simulink model "Frida"  (R2024b)
settings: Solver=VariableStepAuto  StartTime=0.0  StopTime=10.0  RelTol=1e-3
settings DataIOCC: SaveTime=off  ReturnWorkspaceOutputs=off  TimeSaveName=t

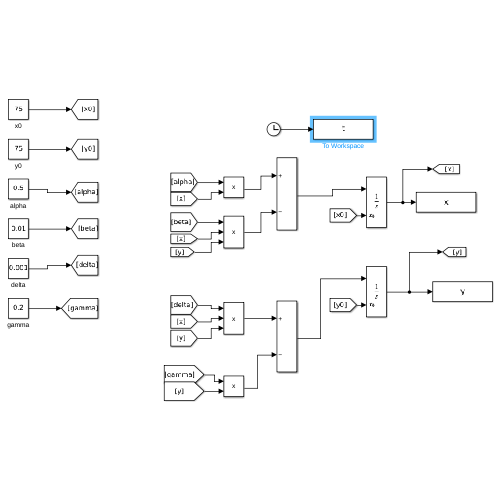
[thumbnail: Simulink's stored preview of the top-level diagram]
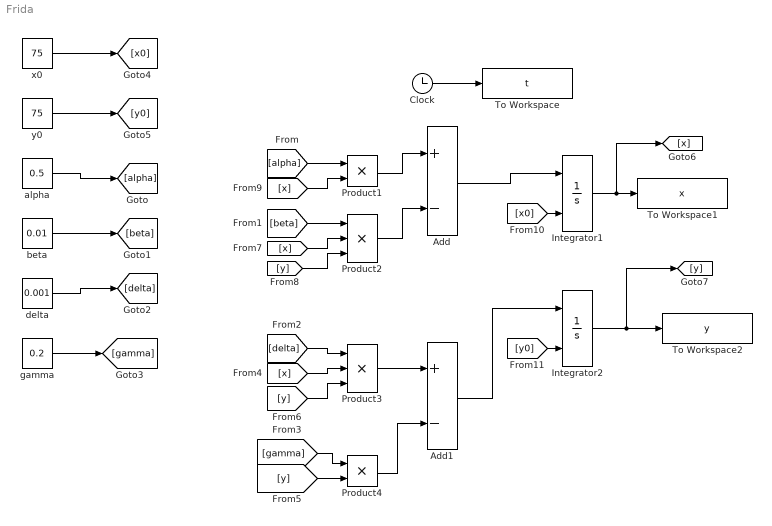
== system Frida ==
  Add : Sum  Inputs=+-
  Add1 : Sum  Inputs=+-
  Clock : Clock
  Integrator1 : Integrator  InitialConditionSource=external
  Integrator2 : Integrator  InitialConditionSource=external
  Product1 : Product
  Product2 : Product  Inputs=3
  Product3 : Product  Inputs=3
  Product4 : Product
  To Workspace : ToWorkspace  VariableName=t  SampleTime=-1
  To Workspace1 : ToWorkspace  VariableName=x  SampleTime=-1
  To Workspace2 : ToWorkspace  VariableName=y  SampleTime=-1
  alpha : Constant  Value=0.5
  beta : Constant  Value=0.01
  delta : Constant  Value=0.001
  gamma : Constant  Value=0.2
  x0 : Constant  Value=75
  y0 : Constant  Value=75
  wires:
  alpha/1 -> [alpha]
  beta/1 -> [beta]
  delta/1 -> [delta]
  gamma/1 -> [gamma]
  Product3/1 -> Add1/1
  Product4/1 -> Add1/2
  Add/1 -> Integrator1/1
  Add1/1 -> Integrator2/1
  [alpha] -> Product1/1
  [beta] -> Product2/1
  [delta] -> Product3/1
  [gamma] -> Product4/1
  x0/1 -> [x0]
  y0/1 -> [y0]
  [y] -> Product4/2
  [x] -> Product3/2
  [y] -> Product3/3
  [x] -> Product2/2
  [y] -> Product2/3
  [x] -> Product1/2
  Product1/1 -> Add/1
  Product2/1 -> Add/2
  [x0] -> Integrator1/2
  [y0] -> Integrator2/2
  Integrator1/1 -> [x], To Workspace1/1
  Integrator2/1 -> [y], To Workspace2/1
  Clock/1 -> To Workspace/1
